simulink model "System"  (R2018a)
settings: Solver=VariableStepAuto  StartTime=0.0  StopTime=Simulation_Runtime  RelTol=1e-3
InitFcn:
  | System_Paramaters
values from neighbouring files (symbols this model uses):
  Fs = 10E3    (= 10000)    [System_Paramaters.m]
libraries: simulink_extras x1
settings Model: Creator=David  LastModifiedBy=David

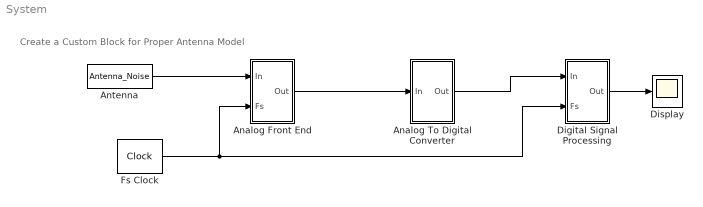
== system System ==
  note: Create a Custom Block for Proper Antenna Model
  Analog Front End : Subsystem
  Analog To Digital Converter : Subsystem
  Antenna : FromWorkspace  VariableName=Antenna_Noise  OutDataTypeStr=double  SampleTime=0  Interpolate=off  OutputAfterFinalValue=Holding final value
  Digital Signal Processing : Subsystem
  Display : Scope
  Fs Clock : simulink_extras/Flip Flops/Clock  period=1/Fs
  wires:
  Antenna/1 -> Analog Front End/1("In ")
  Analog Front End/1(Out) -> Analog To Digital Converter/1(In)
  Analog To Digital Converter/1(Out) -> Digital Signal Processing/1(In)
  Digital Signal Processing/1(Out) -> Display/1
  Fs Clock/1 -> Analog Front End/2(Fs), Digital Signal Processing/2(Fs)

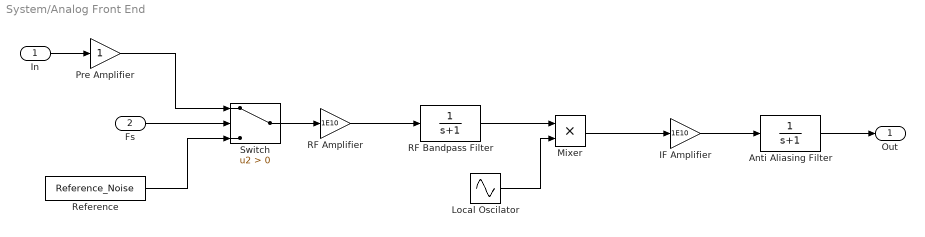
== system System/Analog Front End ==
  "In " : Inport
  Fs : Inport  Port=2
  Anti Aliasing Filter : TransferFcn  Denominator=[1 1]
  IF Amplifier : Gain  Gain=1E10
  Local Oscilator : Sin  SampleTime=0
  Mixer : Product
  Pre Amplifier : Gain
  RF Amplifier : Gain  Gain=1E10
  RF Bandpass Filter : TransferFcn  Denominator=[1 1]
  Reference : FromWorkspace  VariableName=Reference_Noise  OutDataTypeStr=double  SampleTime=0  Interpolate=off  OutputAfterFinalValue=Holding final value
  Switch : Switch  Criteria=u2 > Threshold
  Out : Outport
  wires:
  Fs/1 -> Switch/2
  Reference/1 -> Switch/3
  "In "/1 -> Pre Amplifier/1
  Pre Amplifier/1 -> Switch/1
  Switch/1 -> RF Amplifier/1
  Local Oscilator/1 -> Mixer/2
  Mixer/1 -> IF Amplifier/1
  RF Bandpass Filter/1 -> Mixer/1
  RF Amplifier/1 -> RF Bandpass Filter/1
  IF Amplifier/1 -> Anti Aliasing Filter/1
  Anti Aliasing Filter/1 -> Out/1

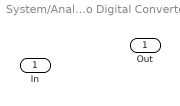
== system System/Analog To Digital Converter ==
  In : Inport
  Out : Outport

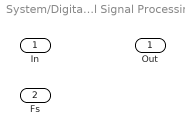
== system System/Digital Signal Processing ==
  In : Inport
  Fs : Inport  Port=2
  Out : Outport
